simulink model "abs_CS9_LDM_w_EBRDBR"  (Simulink 9.2)
settings: Solver=FixedStepAuto  StartTime=0  StopTime=20  FixedStep=0.0005  RelTol=1e-3  AbsTol=1e-6
values from neighbouring files (symbols this model uses):
  K_Cntr_HiSpd_u8 = 10.0    [DBR_V002.sldd]
  K_Cntr_LowSpd_u8 = 10.0    [DBR_V002.sldd]
  K_Cntr_NrmlSpd_u8 = 10.0    [DBR_V002.sldd]
  K_Cntr_Sdstl_u8 = 10.0    [DBR_V002.sldd]
  K_CSTCtol_ramp_lower = -800.0    [DBR_V002.sldd]
  K_CSTCtol_ramp_upper = 800.0    [DBR_V002.sldd]
  K_DBR_aDBRCSTminDecel = 100.0    [DBR_V002.sldd]
  K_DBR_aDBRDecelEmgHigh_CST_u16 = 500.0    [DBR_V002.sldd]
  K_DBR_aDBRDecelSftLow_CST_u16 = 200.0    [DBR_V002.sldd]
  K_DBR_aDBRDecelStdlstlDegdlvl1_u16 = 600.0    [DBR_V002.sldd]
  K_DBR_aDBRDecelStdlstlDegdlvl2_u16 = 1200.0    [DBR_V002.sldd]
  K_DBR_blCSTSwch_bl = 0.0    [DBR_V002.sldd]
  K_DBR_coDBRDecelFactor1 = 5.0    [DBR_V002.sldd]
  K_DBR_coDBRDecelFactor2 = 3.0    [DBR_V002.sldd]
  K_DBR_lenDBRStdlstlDegdlvl_u16 = 1800.0    [DBR_V002.sldd]
  K_DBR_velCSTPdlDistSpdLmt_s16 = 100.0    [DBR_V002.sldd]
  K_DBR_velDBRCSTlowVehSpd_u16 = 8.0    [DBR_V002.sldd]
  K_DBR_velVehSpdLow_CST_s16 = 14.0    [DBR_V002.sldd]
  K_EBR_aACCHold_flat_u16 = 200.0    [DBR_V002.sldd]
  K_EBR_ACC_ramp_lower = -800.0    [DBR_V002.sldd]
  K_EBR_ACC_ramp_upper = 800.0    [DBR_V002.sldd]
  K_EBR_ACCSBDeclEterDecl_u16 = 200.0    [DBR_V002.sldd]
  K_EBR_ACCSBDeclSlope = 1.0    [DBR_V002.sldd]
  K_EBR_ACCSBminDecl = 100.0    [DBR_V002.sldd]
  K_EBR_velACCVehSpdHiLim_u16 = 431.0    [DBR_V002.sldd]
  K_EBR_velACCVehSpdLim_buffer = 1.0    [DBR_V002.sldd]
  K_EBR_velACCVehSpdLoLim_u16 = 14.0    [DBR_V002.sldd]
  W_EBR_velACCSBEntrVehSpd_u16 = 0.0    [DBR_V002.sldd]
undefined symbols (not defined in the file or in its folder): sigbuilder_block
libraries: simulink x8, LDM_Controller x2, Solver_SF x1
(part 1 of 2)
settings Model: DataDictionary=totalDataDict.sldd  Creator=ywata  LastModifiedBy=wxmjy  PauseTimes=12.5  NumberOfSteps=10  ExtModeTrigMode=oneshot  ExtModeArmWhenConnect=off
settings SolverCC: AutoScaleAbsTol=off
settings DataIOCC: LimitDataPoints=off  SaveFormat=Dataset  SignalLoggingSaveFormat=Dataset  SignalLoggingName=sigsOut
settings OptimizationCC: BlockReduction=off  BooleanDataType=off  ExpressionDepthLimit=2147483647
settings DebuggingCC: SaveWithParameterizedLinksMsg=none  SignalResolutionControl=TryResolveAllWithWarning  MultiTaskDSMMsg=warning  MultiTaskCondExecSysMsg=none
settings HardwareCC: TargetUnknown=on
settings RTWCC: TemplateMakefile=grt_vc.tmf
settings GRTTargetCC: TargetFcnLib=ansi_tfl_tmw.mat  GeneratePreprocessorConditionals=Use local settings
settings ConfigComp: CovHtmlReporting=off

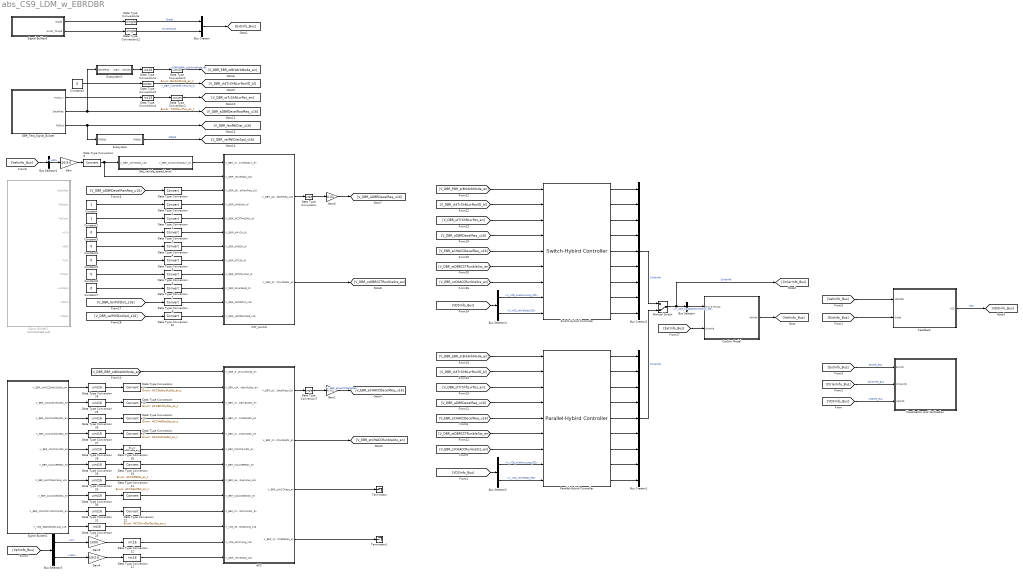
== system abs_CS9_LDM_w_EBRDBR ==
  ACC : Subsystem
  Bus Creator : BusCreator  Inputs=2
  Bus Creator1 : BusCreator  Inputs=9
  Bus Creator2 : BusCreator  Inputs=9
  Bus Selector : BusSelector  OutputSignals=V_LDM_torqDecelCtrlerOut_f32
  Bus Selector1 : BusSelector  OutputSignals=xdot
  Bus Selector2 : BusSelector  OutputSignals=V_VDS_aVehAccLong_f32,V_VDS_velVehSpd_f32
  Bus Selector3 : BusSelector  OutputSignals=ax,xdot
  Bus Selector4 : BusSelector  OutputSignals=V_VDS_aVehAccLong_f32,V_VDS_velVehSpd_f32
  CST_control : Subsystem
  CarSim Model : Subsystem
  Constant : Constant
  Constant1 : Constant
  Constant{2..7} (6 alike) : Constant  Value=0
  DBR_Test_Signal_Builder : Subsystem  Tag=STV Subsys  LoadFcn=sigbuilder_block('load',[245.25 59.25 620.25 643.5 ]);  StartFcn=sigbuilder_block('start');  StopFcn=sigbuilder_block('stop');  ClipboardFcn=sigbuilder_block('clipboard');  mask(Sigbuilder block){tuvar=[0:10]}
      mask help: Simulink:masks:SigbuilderBlock_MD
      mask init:
      | if ~strcmp(get_param(bdroot(gcbh),'SimulationStatus'),'stopped') tuvar = sigbuilder_block('maskInit'); end
      settings: CopyFcn=sigbuilder_block('copy');  DeleteFcn=sigbuilder_block('delete');  ModelCloseFcn=sigbuilder_block('modelClose');  PreSaveFcn=sigbuilder_block('preSave');  PauseFcn=sigbuilder_block('pause');  ContinueFcn=sigbuilder_block('continue');  NameChangeFcn=sigbuilder_block('namechange');  OpenFcn=sigbuilder_block('open',[782.25 67.5 620.25 643.5 ]);  CloseFcn=sigbuilder_block('close');
      mask Display: plot(0, 0, 100, 100,[2, 2, 32, 32, 2], [68, 8, 8, 68, 68],[32, 2], [38, 38], [32, 19, 2],[53, 60, 44], [32, 17, 17, 2],[16, 16, 31, 31]);txt = getActiveGroup(gcbh);text(2, 100, txt,'verticalAlignment', 'top');
  Data Type  Conversion{,6..7,12} (4 alike) : DataTypeConversion  OutDataTypeStr=single
  Data Type  Conversion1 : DataTypeConversion  OutDataTypeStr=Enum: BrkArbMode_en_t
  Data Type  Conversion2 : DataTypeConversion  OutDataTypeStr=Enum: TrShftLvrPos_en_t
  Data Type  Conversion3 : DataTypeConversion  OutDataTypeStr=int16
  Data Type  Conversion4 : DataTypeConversion  OutDataTypeStr=int16
  Data Type  Conversion5 : DataTypeConversion  OutDataTypeStr=boolean  RndMeth=Nearest
  Data Type Conversion{,1..8,32} (10 alike) : DataTypeConversion
  Data Type Conversion11 : DataTypeConversion  OutDataTypeStr=int16  RndMeth=Ceiling
  Data Type Conversion12 : DataTypeConversion  OutDataTypeStr=int16  RndMeth=Ceiling
  Data Type Conversion14 : DataTypeConversion  OutDataTypeStr=Enum: ACCStdbySkpSts_en_t
  Data Type Conversion15 : DataTypeConversion  OutDataTypeStr=Enum: ACCBrkSkpSts_en_t
  Data Type Conversion16 : DataTypeConversion  OutDataTypeStr=Enum: ACCHldSkpSts_en_t
  Data Type Conversion17 : DataTypeConversion  OutDataTypeStr=Enum: ACCFalCseSts_en_t
  Data Type Conversion18 : DataTypeConversion  OutDataTypeStr=Enum: ACCSysSts_en_t
  Data Type Conversion19 : DataTypeConversion  OutDataTypeStr=Enum: ACCEPBSts_en_t
  Data Type Conversion{20,24..31} (9 alike) : DataTypeConversion  OutDataTypeStr=uint16
  Data Type Conversion21 : DataTypeConversion  OutDataTypeStr=Enum: ACCSebltSts_en_t
  Data Type Conversion22 : DataTypeConversion  OutDataTypeStr=Enum: ACCDrvrDorOpnSts_en_t
  Data Type Conversion23 : DataTypeConversion  OutDataTypeStr=int16
  Data Type Conversion9 : DataTypeConversion  RndMeth=Ceiling
  Feedback : Subsystem
  Gain : Gain  Gain=10/3.6
  Gain1 : Gain  Gain=0.01  OutDataTypeStr=Inherit: Inherit via back propagation
  Gain4 : Gain  Gain=10/3.6
  Gain5 : Gain  Gain=1000
  Gain6 : Gain  Gain=0.01  OutDataTypeStr=Inherit: Inherit via back propagation
  Get_vehicle_speed_level : Subsystem
  Manual Switch : ManualSwitch  CurrentSetting=0
  Parallel-Hybird Controller : LDM_Controller/Parallel-Hybird Controller  SystemSampleTime=-1
  Signal Builder1 : Subsystem  Tag=STV Subsys  Commented=on  LoadFcn=sigbuilder_block('load');  StartFcn=sigbuilder_block('start');  StopFcn=sigbuilder_block('stop');  ClipboardFcn=sigbuilder_block('clipboard');  mask(Sigbuilder block){tuvar=[0:10]}
      mask help: Simulink:masks:SigbuilderBlock_MD
      mask init:
      | if ~strcmp(get_param(bdroot(gcbh),'SimulationStatus'),'stopped') tuvar = sigbuilder_block('maskInit'); end
      settings: CopyFcn=sigbuilder_block('copy');  DeleteFcn=sigbuilder_block('delete');  ModelCloseFcn=sigbuilder_block('modelClose');  PreSaveFcn=sigbuilder_block('preSave');  PauseFcn=sigbuilder_block('pause');  ContinueFcn=sigbuilder_block('continue');  NameChangeFcn=sigbuilder_block('namechange');  OpenFcn=sigbuilder_block('open',[0.75 30.75 718.5 714.75 ]);  CloseFcn=sigbuilder_block('close');
      mask Display: plot(0, 0, 100, 100,[2, 2, 32, 32, 2], [68, 8, 8, 68, 68],[32, 2], [38, 38], [32, 19, 2],[53, 60, 44], [32, 17, 17, 2],[16, 16, 31, 31]);txt = getActiveGroup(gcbh);text(2, 100, txt,'verticalAlignment', 'top');
  Signal Builder2 : Subsystem  Tag=STV Subsys  LoadFcn=sigbuilder_block('load');  StartFcn=sigbuilder_block('start');  StopFcn=sigbuilder_block('stop');  ClipboardFcn=sigbuilder_block('clipboard');  mask(Sigbuilder block){tuvar=[0:10]}
      mask help: Simulink:masks:SigbuilderBlock_MD
      mask init:
      | if ~strcmp(get_param(bdroot(gcbh),'SimulationStatus'),'stopped') tuvar = sigbuilder_block('maskInit'); end
      settings: CopyFcn=sigbuilder_block('copy');  DeleteFcn=sigbuilder_block('delete');  ModelCloseFcn=sigbuilder_block('modelClose');  PreSaveFcn=sigbuilder_block('preSave');  PauseFcn=sigbuilder_block('pause');  ContinueFcn=sigbuilder_block('continue');  NameChangeFcn=sigbuilder_block('namechange');  OpenFcn=sigbuilder_block('open',[0.75 30.75 718.5 714.75 ]);  CloseFcn=sigbuilder_block('close');
      mask Display: plot(0, 0, 100, 100,[2, 2, 32, 32, 2], [68, 8, 8, 68, 68],[32, 2], [38, 38], [32, 19, 2],[53, 60, 44], [32, 17, 17, 2],[16, 16, 31, 31]);txt = getActiveGroup(gcbh);text(2, 100, txt,'verticalAlignment', 'top');
  Signal Builder3 : Subsystem  Tag=STV Subsys  LoadFcn=sigbuilder_block('load');  StartFcn=sigbuilder_block('start');  StopFcn=sigbuilder_block('stop');  ClipboardFcn=sigbuilder_block('clipboard');  mask(Sigbuilder block){tuvar=[0:10]}
      mask help: Simulink:masks:SigbuilderBlock_MD
      mask init:
      | if ~strcmp(get_param(bdroot(gcbh),'SimulationStatus'),'stopped') tuvar = sigbuilder_block('maskInit'); end
      settings: CopyFcn=sigbuilder_block('copy');  DeleteFcn=sigbuilder_block('delete');  ModelCloseFcn=sigbuilder_block('modelClose');  PreSaveFcn=sigbuilder_block('preSave');  PauseFcn=sigbuilder_block('pause');  ContinueFcn=sigbuilder_block('continue');  NameChangeFcn=sigbuilder_block('namechange');  OpenFcn=sigbuilder_block('open',[782.25 67.5 620.25 643.5 ]);  CloseFcn=sigbuilder_block('close');
      mask Display: plot(0, 0, 100, 100,[2, 2, 32, 32, 2], [68, 8, 8, 68, 68],[32, 2], [38, 38], [32, 19, 2],[53, 60, 44], [32, 17, 17, 2],[16, 16, 31, 31]);txt = getActiveGroup(gcbh);text(2, 100, txt,'verticalAlignment', 'top');
  Subsystem : Subsystem
  Subsystem1 : Subsystem
  Switch-Hybird Controller : LDM_Controller/Switch-Hybird Controller  SystemSampleTime=-1
  Terminator : Terminator
  Terminator1 : Terminator
  Visualization and Verification : Subsystem
  wires:
  [ExtInfo_Bus] -> Visualization and Verification/1(ExtInfo)  "ExtInfo_Bus"
  [V_EBR_aCHACCDecelReq_u16] -> Parallel-Hybird Controller/5
  Data Type  Conversion12/1 -> Bus Creator/2  "DriveTorque"
  Data Type  Conversion3/1 -> Data Type  Conversion1/1
  Data Type  Conversion4/1 -> Data Type  Conversion2/1
  [V_EBR_stCHACCRunbleSts_en] -> Parallel-Hybird Controller/7
  Constant2/1 -> Data Type  Conversion5/1
  Data Type  Conversion6/1 -> Bus Creator/1  "Grade"
  Subsystem1/1(stBrkArbMode) -> Data Type  Conversion3/1
  Data Type  Conversion1/1 -> [V_DBR_EBR_stBrkArbMode_en]  "V_DBR_EBR_stBrkArbMode_en"
  DBR_Test_Signal_Builder/1(TrShtLvr) -> Data Type  Conversion4/1
  Data Type  Conversion2/1 -> [V_DBR_stTrShftLvrPos_en]
  Feedback/1(VDS) -> [VDSInfo_Bus]  "VDS"
  Signal Builder3/2(Accel_Torque) -> Data Type  Conversion12/1
  [CtrlerInfo_Bus] -> Visualization and Verification/2(CtrlerInfo)  "CtrlerInfo_Bus"
  Data Type  Conversion5/1 -> [V_DBR_vldTrShftLvrPosVD_bl]  "V_DBR_vldTrShftLvrPosVD_bl"
  [VehInfo_Bus] -> Feedback/1(VehFdbk)
  CarSim Model/1(VehInfo) -> [VehInfo_Bus]
  Bus Creator/1 -> [ExtInfo_Bus]
  Manual Switch/1 -> [CtrlerInfo_Bus], Bus Selector/1  "CtrlerInfo"
  [VDSInfo_Bus] -> Visualization and Verification/3(VehInfo)  "VDSInfo_Bus"
  [ExtInfo_Bus] -> Feedback/2(Grade)
  Bus Selector1/1 -> Gain/1  "<xdot>"
  Get_vehicle_speed_level/1(V_EBR_stACCVehSpdLvl_en) -> CST_control/1(V_EBR_stACCVehSpdLvl_en)
  [V_DBR_aDBRDecelRawReq_u16] -> Data Type Conversion/1
  Constant/1 -> Data Type Conversion1/1
  Constant1/1 -> Data Type Conversion2/1
  Constant3/1 -> Data Type Conversion3/1
  Constant4/1 -> Data Type Conversion4/1
  Constant5/1 -> Data Type Conversion5/1
  Constant6/1 -> Data Type Conversion6/1
  Constant7/1 -> Data Type Conversion7/1
  [VehInfo_Bus] -> Bus Selector1/1
  Data Type Conversion/1 -> CST_control/3(V_DBR_aDBRDecelRawReq_u16)
  Data Type Conversion1/1 -> CST_control/4(V_DBR_stPdlAply_bl)
  Data Type Conversion2/1 -> CST_control/5(V_DBR_blCSTPreCdtin_bl)
  Data Type Conversion3/1 -> CST_control/6(V_DBR_blAYCA_bl)
  Data Type Conversion4/1 -> CST_control/7(V_DBR_blABSA_bl)
  Data Type Conversion5/1 -> CST_control/8(V_DBR_blTCSA_bl)
  Data Type Conversion6/1 -> CST_control/9(V_DBR_blCSTSysFail_bl)
  Data Type Conversion7/1 -> CST_control/10(V_DBR_blLosDecel_bl)
  Data Type Conversion8/1 -> CST_control/11(V_DBR_lenPdlDist_s16)
  Data Type Conversion9/1 -> CST_control/2(V_DBR_velVehSpd_s16), Get_vehicle_speed_level/1(V_DBR_velVehSpd_s16)
  Gain/1 -> Data Type Conversion9/1
  Gain6/1 -> [V_DBR_aDBRDecelReq_u16]
  CST_control/2(V_DBR_stDBRCSTRunbleSts_en) -> [V_DBR_stDBRCSTRunbleSts_en]
  ACC/3(V_EBR_stACCResp_en) -> Terminator/1
  Data Type Conversion11/1 -> ACC/13(V_DBR_velVehSpd_s16)
  ACC/4(V_EBR_stCHACCEPBReq_en) -> Terminator1/1
  [V_DBR_EBR_stBrkArbMode_en] -> ACC/1(V_DBR_EBR_stBrkArbMode_en)
  Gain4/1 -> Data Type Conversion11/1
  [VehInfo_Bus] -> Bus Selector3/1
  Bus Selector3/2 -> Gain4/1  "<xdot>"
  Bus Selector3/1 -> Gain5/1  "<ax>"
  Gain5/1 -> Data Type Conversion12/1
  Data Type Conversion12/1 -> ACC/12(V_VDS_aACCLong_s16)
  ACC/2(V_EBR_stCHACCRunbleSts_en) -> [V_EBR_stCHACCRunbleSts_en]
  Signal Builder2/1(V_EBR_stACCStdbySkpSts_en) -> Data Type Conversion24/1
  Signal Builder2/2(V_EBR_stACCBrkSkpSts_en) -> Data Type Conversion25/1
  Signal Builder2/3(V_EBR_stACCHldSkpSts_en) -> Data Type Conversion26/1
  Signal Builder2/4(V_EBR_stACCFalCseSts_en) -> Data Type Conversion27/1
  Signal Builder2/5(V_EBR_stACCSysSts_en) -> Data Type Conversion28/1
  Signal Builder2/6(V_EBR_stACCEPBSts_en) -> Data Type Conversion29/1
  Signal Builder2/7(V_EBR_aACCReqValue_u16) -> Data Type Conversion20/1
  Signal Builder2/8(V_EBR_stACCSebltSts_en) -> Data Type Conversion30/1
  Signal Builder2/9(V_EBR_stACCDrvrDorOpnSts_en) -> Data Type Conversion31/1
  Signal Builder2/10(V_VDS_degRdSlopeLong_s16) -> Data Type Conversion23/1
  Data Type Conversion14/1 -> ACC/2(V_EBR_stACCStdbySkpSts_en)
  Data Type Conversion15/1 -> ACC/3(V_EBR_stACCBrkSkpSts_en)
  Data Type Conversion16/1 -> ACC/4(V_EBR_stACCHldSkpSts_en)
  Data Type Conversion17/1 -> ACC/5(V_EBR_stACCFalCseSts_en)
  Data Type Conversion18/1 -> ACC/6(V_EBR_stACCSysSts_en)
  Data Type Conversion19/1 -> ACC/7(V_EBR_stACCEPBSts_en)
  Data Type Conversion20/1 -> ACC/8(V_EBR_aACCReqValue_u16)
  Data Type Conversion21/1 -> ACC/9(V_EBR_stACCSebltSts_en)
  Data Type Conversion22/1 -> ACC/10(V_EBR_stACCDrvrDorOpnSts_en)
  Data Type Conversion23/1 -> ACC/11(V_VDS_degRdSlopeLong_s16)
  Data Type Conversion24/1 -> Data Type Conversion14/1
  Data Type Conversion25/1 -> Data Type Conversion15/1
  Data Type Conversion26/1 -> Data Type Conversion16/1
  Data Type Conversion27/1 -> Data Type Conversion17/1
  Data Type Conversion28/1 -> Data Type Conversion18/1
  Data Type Conversion29/1 -> Data Type Conversion19/1
  Data Type Conversion30/1 -> Data Type Conversion21/1
  Data Type Conversion31/1 -> Data Type Conversion22/1
  Data Type Conversion32/1 -> CST_control/12(V_DBR_velPdlDistSpd_s16)
  [V_DBR_aDBRDecelReq_u16] -> Parallel-Hybird Controller/4
  [V_DBR_stDBRCSTRunbleSts_en] -> Parallel-Hybird Controller/6
  [V_DBR_EBR_stBrkArbMode_en] -> Parallel-Hybird Controller/1
  [V_DBR_vldTrShftLvrPosVD_bl] -> Parallel-Hybird Controller/2
  [V_DBR_stTrShftLvrPos_en] -> Parallel-Hybird Controller/3
  Bus Selector/1 -> CarSim Model/1(Brake Torque)  "<V_LDM_torqDecelCtrlerOut_f32>"
  DBR_Test_Signal_Builder/2(DecelReq) -> Subsystem1/1(DecelReq), [V_DBR_aDBRDecelRawReq_u16]
  DBR_Test_Signal_Builder/3(PldDist) -> Subsystem/1(PldDist), [V_DBR_lenPdlDist_s16]
  Subsystem/1(PldSpd) -> [V_DBR_velPdlDistSpd_s16]  "PldSpd"
  [V_DBR_velPdlDistSpd_s16] -> Data Type Conversion32/1
  [V_DBR_lenPdlDist_s16] -> Data Type Conversion8/1
  Signal Builder3/1(Grade) -> Data Type  Conversion6/1
  [VDSInfo_Bus] -> Bus Selector2/1
  Bus Selector2/1 -> Parallel-Hybird Controller/8  "<V_VDS_aVehAccLong_f32>"
  Bus Selector2/2 -> Parallel-Hybird Controller/9  "<V_VDS_velVehSpd_f32>"
  Parallel-Hybird Controller/1 -> Bus Creator1/1
  Parallel-Hybird Controller/2 -> Bus Creator1/2
  Parallel-Hybird Controller/4 -> Bus Creator1/4
  Parallel-Hybird Controller/5 -> Bus Creator1/5
  Parallel-Hybird Controller/6 -> Bus Creator1/6
  Parallel-Hybird Controller/7 -> Bus Creator1/7
  Parallel-Hybird Controller/8 -> Bus Creator1/8
  Bus Selector4/2 -> Switch-Hybird Controller/9  "<V_VDS_velVehSpd_f32>"
  Bus Selector4/1 -> Switch-Hybird Controller/8  "<V_VDS_aVehAccLong_f32>"
  [VDSInfo_Bus] -> Bus Selector4/1
  [V_DBR_stTrShftLvrPos_en] -> Switch-Hybird Controller/3
  [V_DBR_vldTrShftLvrPosVD_bl] -> Switch-Hybird Controller/2
  [V_DBR_EBR_stBrkArbMode_en] -> Switch-Hybird Controller/1
  [V_DBR_stDBRCSTRunbleSts_en] -> Switch-Hybird Controller/6
  [V_DBR_aDBRDecelReq_u16] -> Switch-Hybird Controller/4
  [V_EBR_stCHACCRunbleSts_en] -> Switch-Hybird Controller/7
  [V_EBR_aCHACCDecelReq_u16] -> Switch-Hybird Controller/5
  Switch-Hybird Controller/8 -> Bus Creator2/8
  Switch-Hybird Controller/7 -> Bus Creator2/7
  Switch-Hybird Controller/6 -> Bus Creator2/6
  Switch-Hybird Controller/5 -> Bus Creator2/5
  Switch-Hybird Controller/4 -> Bus Creator2/4
  Switch-Hybird Controller/2 -> Bus Creator2/2
  Switch-Hybird Controller/1 -> Bus Creator2/1
  Bus Creator2/1 -> Manual Switch/1  "CtrlerInfo"
  Bus Creator1/1 -> Manual Switch/2  "CtrlerInfo"
  Switch-Hybird Controller/9 -> Bus Creator2/9
  Parallel-Hybird Controller/9 -> Bus Creator1/9
  [ExtInfo_Bus] -> CarSim Model/2(throttle)
  Parallel-Hybird Controller/3 -> Bus Creator1/3
  Switch-Hybird Controller/3 -> Bus Creator2/3
  Data Type  Conversion7/1 -> Gain1/1
  Data Type  Conversion/1 -> Gain6/1
  CST_control/1(V_DBR_aDBRDecelReq_u16) -> Data Type  Conversion/1
  Gain1/1 -> [V_EBR_aCHACCDecelReq_u16]  "V_EBR_aCHACCDecelReq"
  ACC/1(V_EBR_aCHACCDecelReq_u16) -> Data Type  Conversion7/1

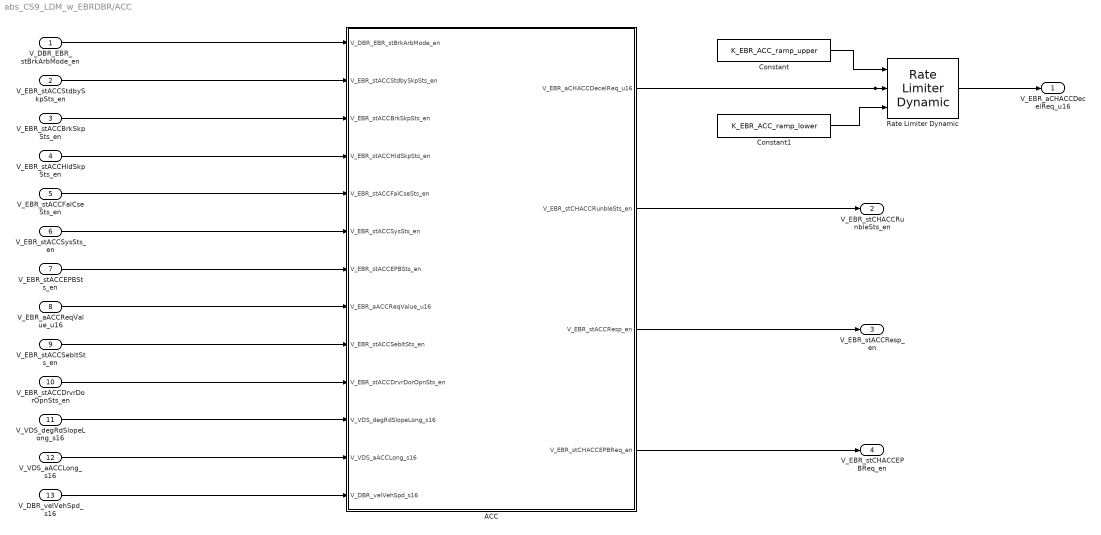
== system abs_CS9_LDM_w_EBRDBR/ACC ==
  V_DBR_EBR_stBrkArbMode_en : Inport
  V_EBR_stACCStdbySkpSts_en : Inport  Port=2
  V_EBR_stACCBrkSkpSts_en : Inport  Port=3
  V_EBR_stACCHldSkpSts_en : Inport  Port=4
  V_EBR_stACCFalCseSts_en : Inport  Port=5
  V_EBR_stACCSysSts_en : Inport  Port=6
  V_EBR_stACCEPBSts_en : Inport  Port=7
  V_EBR_aACCReqValue_u16 : Inport  Port=8
  V_EBR_stACCSebltSts_en : Inport  Port=9
  V_EBR_stACCDrvrDorOpnSts_en : Inport  Port=10
  V_VDS_degRdSlopeLong_s16 : Inport  Port=11
  V_VDS_aACCLong_s16 : Inport  Port=12
  V_DBR_velVehSpd_s16 : Inport  Port=13
  ACC : Stateflow chart  TreatAsAtomicUnit=on
  Constant : Constant  Value=K_EBR_ACC_ramp_upper
  Constant1 : Constant  Value=K_EBR_ACC_ramp_lower
  Rate Limiter Dynamic : simulink/Discontinuities/Rate Limiter Dynamic
      settings: SourceProductName=Simulink
  V_EBR_aCHACCDecelReq_u16 : Outport
  V_EBR_stCHACCRunbleSts_en : Outport  Port=2  OutDataTypeStr=Enum: CHACCRunbleSts_en_t
  V_EBR_stACCResp_en : Outport  Port=3  OutDataTypeStr=Enum: ACCResp_en_t
  V_EBR_stCHACCEPBReq_en : Outport  Port=4  OutDataTypeStr=Enum: CHACCEPBReq_en_t
  wires:
  V_EBR_stACCStdbySkpSts_en/1 -> ACC/2(V_EBR_stACCStdbySkpSts_en)
  V_EBR_stACCBrkSkpSts_en/1 -> ACC/3(V_EBR_stACCBrkSkpSts_en)
  V_EBR_stACCHldSkpSts_en/1 -> ACC/4(V_EBR_stACCHldSkpSts_en)
  V_EBR_stACCFalCseSts_en/1 -> ACC/5(V_EBR_stACCFalCseSts_en)
  V_EBR_stACCSysSts_en/1 -> ACC/6(V_EBR_stACCSysSts_en)
  V_EBR_stACCEPBSts_en/1 -> ACC/7(V_EBR_stACCEPBSts_en)
  V_EBR_aACCReqValue_u16/1 -> ACC/8(V_EBR_aACCReqValue_u16)
  V_DBR_EBR_stBrkArbMode_en/1 -> ACC/1(V_DBR_EBR_stBrkArbMode_en)
  V_EBR_stACCSebltSts_en/1 -> ACC/9(V_EBR_stACCSebltSts_en)
  V_EBR_stACCDrvrDorOpnSts_en/1 -> ACC/10(V_EBR_stACCDrvrDorOpnSts_en)
  V_VDS_degRdSlopeLong_s16/1 -> ACC/11(V_VDS_degRdSlopeLong_s16)
  V_VDS_aACCLong_s16/1 -> ACC/12(V_VDS_aACCLong_s16)
  V_DBR_velVehSpd_s16/1 -> ACC/13(V_DBR_velVehSpd_s16)
  ACC/2(V_EBR_stCHACCRunbleSts_en) -> V_EBR_stCHACCRunbleSts_en/1
  ACC/3(V_EBR_stACCResp_en) -> V_EBR_stACCResp_en/1
  ACC/4(V_EBR_stCHACCEPBReq_en) -> V_EBR_stCHACCEPBReq_en/1
  Constant1/1 -> Rate Limiter Dynamic/3
  Constant/1 -> Rate Limiter Dynamic/1
  ACC/1(V_EBR_aCHACCDecelReq_u16) -> Rate Limiter Dynamic/2, V_EBR_aCHACCDecelReq_u16/1

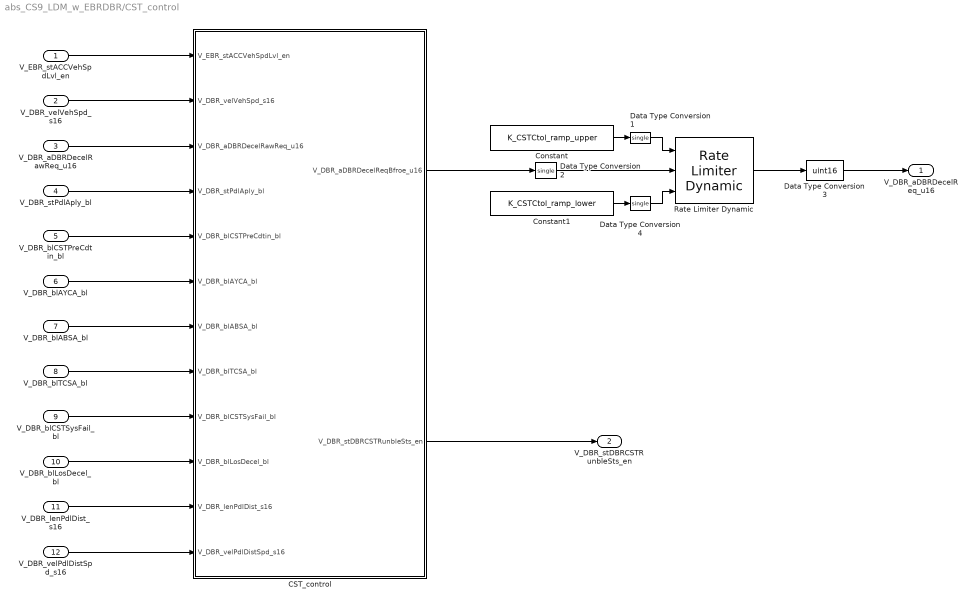
== system abs_CS9_LDM_w_EBRDBR/CST_control ==
  V_EBR_stACCVehSpdLvl_en : Inport
  V_DBR_velVehSpd_s16 : Inport  Port=2
  V_DBR_aDBRDecelRawReq_u16 : Inport  Port=3
  V_DBR_stPdlAply_bl : Inport  Port=4
  V_DBR_blCSTPreCdtin_bl : Inport  Port=5
  V_DBR_blAYCA_bl : Inport  Port=6
  V_DBR_blABSA_bl : Inport  Port=7
  V_DBR_blTCSA_bl : Inport  Port=8
  V_DBR_blCSTSysFail_bl : Inport  Port=9
  V_DBR_blLosDecel_bl : Inport  Port=10
  V_DBR_lenPdlDist_s16 : Inport  Port=11
  V_DBR_velPdlDistSpd_s16 : Inport  Port=12
  CST_control : Stateflow chart  TreatAsAtomicUnit=on
  Constant : Constant  Value=K_CSTCtol_ramp_upper
  Constant1 : Constant  Value=K_CSTCtol_ramp_lower
  Data Type Conversion1 : DataTypeConversion  OutDataTypeStr=single
  Data Type Conversion2 : DataTypeConversion  OutDataTypeStr=single
  Data Type Conversion3 : DataTypeConversion  OutDataTypeStr=uint16
  Data Type Conversion4 : DataTypeConversion  OutDataTypeStr=single
  Rate Limiter Dynamic : simulink/Discontinuities/Rate Limiter Dynamic
  V_DBR_aDBRDecelReq_u16 : Outport
  V_DBR_stDBRCSTRunbleSts_en : Outport  Port=2
  wires:
  V_EBR_stACCVehSpdLvl_en/1 -> CST_control/1(V_EBR_stACCVehSpdLvl_en)
  V_DBR_velVehSpd_s16/1 -> CST_control/2(V_DBR_velVehSpd_s16)
  V_DBR_aDBRDecelRawReq_u16/1 -> CST_control/3(V_DBR_aDBRDecelRawReq_u16)
  V_DBR_stPdlAply_bl/1 -> CST_control/4(V_DBR_stPdlAply_bl)
  V_DBR_blCSTPreCdtin_bl/1 -> CST_control/5(V_DBR_blCSTPreCdtin_bl)
  V_DBR_blAYCA_bl/1 -> CST_control/6(V_DBR_blAYCA_bl)
  V_DBR_blABSA_bl/1 -> CST_control/7(V_DBR_blABSA_bl)
  V_DBR_blTCSA_bl/1 -> CST_control/8(V_DBR_blTCSA_bl)
  V_DBR_blCSTSysFail_bl/1 -> CST_control/9(V_DBR_blCSTSysFail_bl)
  V_DBR_blLosDecel_bl/1 -> CST_control/10(V_DBR_blLosDecel_bl)
  V_DBR_lenPdlDist_s16/1 -> CST_control/11(V_DBR_lenPdlDist_s16)
  CST_control/2(V_DBR_stDBRCSTRunbleSts_en) -> V_DBR_stDBRCSTRunbleSts_en/1
  Rate Limiter Dynamic/1 -> Data Type Conversion3/1
  CST_control/1(V_DBR_aDBRDecelReqBfroe_u16) -> Data Type Conversion2/1
  Data Type Conversion1/1 -> Rate Limiter Dynamic/1
  Data Type Conversion4/1 -> Rate Limiter Dynamic/3
  Data Type Conversion2/1 -> Rate Limiter Dynamic/2
  Constant/1 -> Data Type Conversion1/1
  Constant1/1 -> Data Type Conversion4/1
  Data Type Conversion3/1 -> V_DBR_aDBRDecelReq_u16/1
  V_DBR_velPdlDistSpd_s16/1 -> CST_control/12(V_DBR_velPdlDistSpd_s16)

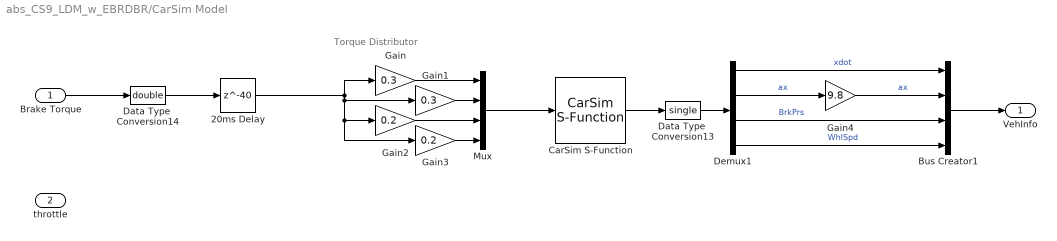
== system abs_CS9_LDM_w_EBRDBR/CarSim Model ==
  note: Torque Distributor
  Brake Torque : Inport
  throttle : Inport  Port=2
  20ms Delay : Delay  DelayLength=40
  Bus Creator1 : BusCreator  Inputs=4
  CarSim S-Function : Solver_SF/CarSim S-Function  Priority=1  SIMFILE=simfile.sim  Run_RTs=off  vs_state_ind=Run  StopMode_ind=Vehicle Model
  Data Type  Conversion13 : DataTypeConversion  OutDataTypeStr=single
  Data Type  Conversion14 : DataTypeConversion  OutDataTypeStr=double
  Demux1 : Demux  Outputs=[1 1 4 4]
  Gain : Gain  Gain=0.3
  Gain1 : Gain  Gain=0.3
  Gain2 : Gain  Gain=0.2
  Gain3 : Gain  Gain=0.2
  Gain4 : Gain  Gain=9.8  OutDataTypeStr=single
  Mux : Mux
  VehInfo : Outport
  wires:
  CarSim S-Function/1 -> Data Type  Conversion13/1
  Bus Creator1/1 -> VehInfo/1
  Demux1/2 -> Gain4/1  "ax"
  Data Type  Conversion13/1 -> Demux1/1
  Demux1/3 -> Bus Creator1/3  "BrkPrs"
  Demux1/4 -> Bus Creator1/4  "WhlSpd"
  Demux1/1 -> Bus Creator1/1  "xdot"
  Brake Torque/1 -> Data Type  Conversion14/1
  Mux/1 -> CarSim S-Function/1
  Gain/1 -> Mux/1
  Gain1/1 -> Mux/2
  Data Type  Conversion14/1 -> 20ms Delay/1
  Gain2/1 -> Mux/3
  Gain3/1 -> Mux/4
  20ms Delay/1 -> Gain3/1, Gain2/1, Gain1/1, Gain/1
  Gain4/1 -> Bus Creator1/2  "ax"

== system abs_CS9_LDM_w_EBRDBR/DBR_Test_Signal_Builder ==
  Demux : Demux  Tag=STV Demux  Outputs=3
  FromWs : FromWorkspace  Tag=STV FromWs  VariableName=tuvar  SampleTime=0  SigBuilderData=DataTag0  VnvData=DataTag1
      SigBuilderData=|
      | common.afterFinalStr = 'Extrapolate'
      | common.sampleTime = 0
      | dataSet(1).timeRange = [0 20]
      | dataSet(1).name = 'DBR_ramp'
      | dataSet(2).timeRange = [0 20]
      | dataSet(2).name = 'DBR_ramp1'
      | dataSet(3).timeRange = [0 20]
      | dataSet(3).name = 'Case1'
      | dataSet(4).timeRange = [0 20]
      | dataSet(4).name = 'Case2'
      | sbobj.Groups(1).Name = 'DBR_ramp'
      | sbobj.Groups(1).Signals(1).Name = 'TrShtLvr'
      | sbobj.Groups(1).Signals(1).XData = [0 20]
      | sbobj.Groups(1).Signals(1).YData = [4 4]
      | sbobj.Groups(1).Signals(2).Name = 'DecelReq'
      | sbobj.Groups(1).Signals(2).XData = [0 4.8 4.8 8.15 8.15 9.85 9.85 14 20]
      | sbobj.Groups(1).Signals(2).YData = [5 5 490 490 180 180 495 0 0]
      | sbobj.Groups(1).Signals(3).Name = 'PldDist'
      | sbobj.Groups(1).Signals(3).XData = [0 2.1 6 10.25 20]
      | sbobj.Groups(1).Signals(3).YData = [0 0 450 0 0]
      | sbobj.Groups(1).TimeRange = [0 20]
      | sbobj.Groups(2).Name = 'DBR_ramp1'
      | sbobj.Groups(2).Signals(1).Name = 'TrShtLvr'
      | sbobj.Groups(2).Signals(1).XData = [0 20]
      | sbobj.Groups(2).Signals(1).YData = [4 4]
      | sbobj.Groups(2).Signals(2).Name = 'DecelReq'
      | sbobj.Groups(2).Signals(2).XData = [0 3.4 3.4 14 14 20]
      | sbobj.Groups(2).Signals(2).YData = [0 0 300 300 20 20]
      | sbobj.Groups(2).Signals(3).Name = 'PldDist'
      | sbobj.Groups(2).Signals(3).XData = [0 20]
      | sbobj.Groups(2).Signals(3).YData = [0 0]
      | sbobj.Groups(2).TimeRange = [0 20]
      | sbobj.Groups(3).Name = 'Case1'
      | sbobj.Groups(3).Signals(1).Name = 'TrShtLvr'
      | sbobj.Groups(3).Signals(1).XData = [0 0.5 3.5 6.5 20]
      | sbobj.Groups(3).Signals(1).YData = [4 4 4 4 4]
      | sbobj.Groups(3).Signals(2).Name = 'DecelReq'
      | sbobj.Groups(3).Signals(2).XData = [0 0.5 3.5 7 12 20]
      | sbobj.Groups(3).Signals(2).YData = [0 0 500 500 0 0]
      | sbobj.Groups(3).Signals(3).Name = 'PldDist'
      | sbobj.Groups(3).Signals(3).XData = [0 0.5 3.5 6.5 20]
      | sbobj.Groups(3).Signals(3).YData = [0 0 50 0 0]
      | sbobj.Groups(3).TimeRange = [0 20]
      | sbobj.Groups(4).Name = 'Case2'
      | sbobj.Groups(4).Signals(1).Name = 'TrShtLvr'
      | sbobj.Groups(4).Signals(1).XData = [0 0.5 1 1.5 20]
      | sbobj.Groups(4).Signals(1).YData = [4 4 4 4 4]
      | sbobj.Groups(4).Signals(2).Name = 'DecelReq'
      | sbobj.Groups(4).Signals(2).XData = [0 0.5 1 1.5 4.9 5.8 7 8.2 9.5 10.35 11.5 12.45 13.7 20]
      | sbobj.Groups(4).Signals(2).YData = [0 0 400 0 0 315 0 0 435 0 0 325 0 0]
      | sbobj.Groups(4).Signals(3).Name = 'PldDist'
      | sbobj.Groups(4).Signals(3).XData = [0 0.5 1 1.5 20]
      | sbobj.Groups(4).Signals(3).YData = [0 0 150 0 0]
      | sbobj.Groups(4).TimeRange = [0 20]
  TrShtLvr : Outport  Tag=STV Outport
  DecelReq : Outport  Tag=STV Outport  Port=2
  PldDist : Outport  Tag=STV Outport  Port=3
  wires:
  FromWs/1 -> Demux/1
  Demux/1 -> TrShtLvr/1
  Demux/2 -> DecelReq/1
  Demux/3 -> PldDist/1

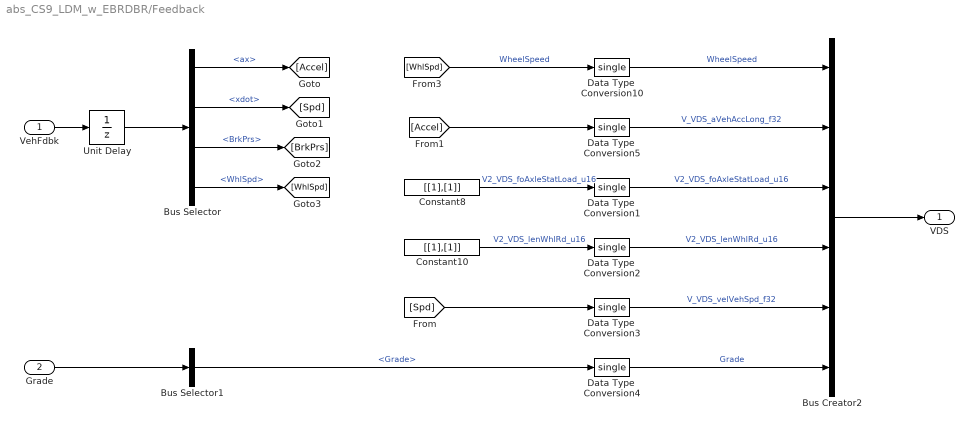
== system abs_CS9_LDM_w_EBRDBR/Feedback ==
  VehFdbk : Inport
  Grade : Inport  Port=2
  Bus Creator2 : BusCreator  Inputs=6
  Bus Selector : BusSelector  OutputSignals=ax,xdot,BrkPrs,WhlSpd
  Bus Selector1 : BusSelector  OutputSignals=Grade
  Constant10 : Constant  Value=[[1],[1]]  OutDataTypeStr=Inherit: Inherit via back propagation
  Constant8 : Constant  Value=[[1],[1]]  OutDataTypeStr=Inherit: Inherit via back propagation
  Data Type  Conversion{1..5,10} (6 alike) : DataTypeConversion  OutDataTypeStr=single
  Unit Delay : UnitDelay  SampleTime=-1
  VDS : Outport
  wires:
  Data Type  Conversion3/1 -> Bus Creator2/5  "V_VDS_velVehSpd_f32"
  Data Type  Conversion10/1 -> Bus Creator2/1  "WheelSpeed"
  Data Type  Conversion2/1 -> Bus Creator2/4  "V2_VDS_lenWhlRd_u16"
  Bus Creator2/1 -> VDS/1
  Data Type  Conversion1/1 -> Bus Creator2/3  "V2_VDS_foAxleStatLoad_u16"
  VehFdbk/1 -> Unit Delay/1
  Bus Selector/1 -> [Accel]  "<ax>"
  Bus Selector/2 -> [Spd]  "<xdot>"
  Bus Selector/3 -> [BrkPrs]  "<BrkPrs>"
  Bus Selector/4 -> [WhlSpd]  "<WhlSpd>"
  Unit Delay/1 -> Bus Selector/1
  Data Type  Conversion4/1 -> Bus Creator2/6  "Grade"
  Constant8/1 -> Data Type  Conversion1/1  "V2_VDS_foAxleStatLoad_u16"
  Constant10/1 -> Data Type  Conversion2/1  "V2_VDS_lenWhlRd_u16"
  Grade/1 -> Bus Selector1/1
  Bus Selector1/1 -> Data Type  Conversion4/1  "<Grade>"
  [WhlSpd] -> Data Type  Conversion10/1  "WheelSpeed"
  [Spd] -> Data Type  Conversion3/1
  [Accel] -> Data Type  Conversion5/1
  Data Type  Conversion5/1 -> Bus Creator2/2  "V_VDS_aVehAccLong_f32"

== system abs_CS9_LDM_w_EBRDBR/Get_vehicle_speed_level ==
  V_DBR_velVehSpd_s16 : Inport  OutDataTypeStr=int16
  Data Type Conversion : DataTypeConversion  OutDataTypeStr=uint16
  Get_vehicle_speed_level : Stateflow chart  TreatAsAtomicUnit=on
  V_EBR_stACCVehSpdLvl_en : Outport
  wires:
  Get_vehicle_speed_level/1(V_EBR_stACCVehSpdLvl_en) -> V_EBR_stACCVehSpdLvl_en/1
  V_DBR_velVehSpd_s16/1 -> Data Type Conversion/1
  Data Type Conversion/1 -> Get_vehicle_speed_level/1(V_DBR_velVehSpd_u16)

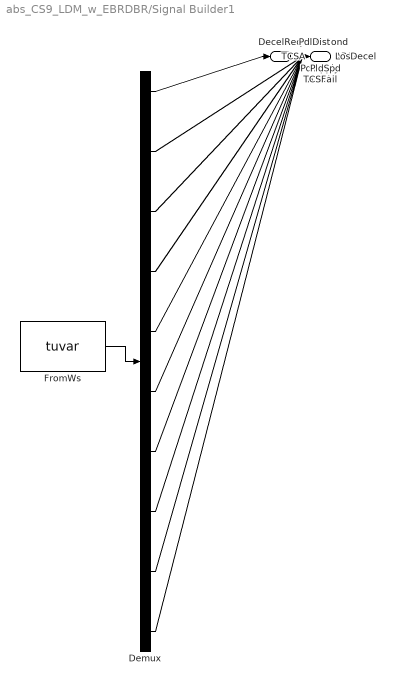
== system abs_CS9_LDM_w_EBRDBR/Signal Builder1 ==
  Demux : Demux  Tag=STV Demux  Outputs=10
  FromWs : FromWorkspace  Tag=STV FromWs  VariableName=tuvar  SampleTime=0  SigBuilderData=DataTag2  VnvData=DataTag3
      SigBuilderData=|
      | common.afterFinalStr = 'Extrapolate'
      | common.sampleTime = 0
      | dataSet.timeRange = [0 20]
      | dataSet.name = 'Group 1'
      | sbobj.Groups.Name = 'Group 1'
      | sbobj.Groups.Signals(1).Name = 'DecelReq'
      | sbobj.Groups.Signals(1).XData = [0 8.1 12 20]
      | sbobj.Groups.Signals(1).YData = [300 370 200 400]
      | sbobj.Groups.Signals(2).Name = 'PdlApply'
      | sbobj.Groups.Signals(2).XData = [0 20]
      | sbobj.Groups.Signals(2).YData = [1 1]
      | sbobj.Groups.Signals(3).Name = 'PreCond'
      | sbobj.Groups.Signals(3).XData = [0 20]
      | sbobj.Groups.Signals(3).YData = [1 1]
      | sbobj.Groups.Signals(4).Name = 'AYCA'
      | sbobj.Groups.Signals(4).XData = [0 20]
      | sbobj.Groups.Signals(4).YData = [0 0]
      | sbobj.Groups.Signals(5).Name = 'ABSA'
      | sbobj.Groups.Signals(5).XData = [0 20]
      | sbobj.Groups.Signals(5).YData = [0 0]
      | sbobj.Groups.Signals(6).Name = 'TCSA'
      | sbobj.Groups.Signals(6).XData = [0 20]
      | sbobj.Groups.Signals(6).YData = [0 0]
      | sbobj.Groups.Signals(7).Name = 'TCSFail'
      | sbobj.Groups.Signals(7).XData = [0 20]
      | sbobj.Groups.Signals(7).YData = [0 0]
      | sbobj.Groups.Signals(8).Name = 'LosDecel'
      | sbobj.Groups.Signals(8).XData = [0 20]
      | sbobj.Groups.Signals(8).YData = [0 0]
      | sbobj.Groups.Signals(9).Name = 'PdlDist'
      | sbobj.Groups.Signals(9).XData = [0 1 5 10 20]
      | sbobj.Groups.Signals(9).YData = [0 0 500 1 1]
      | sbobj.Groups.Signals(10).Name = 'PldSpd'
      | sbobj.Groups.Signals(10).XData = [0 5.4 10 10 20]
      | sbobj.Groups.Signals(10).YData = [0 115 105 1 1]
      | sbobj.Groups.TimeRange = [0 20]
  DecelReq : Outport  Tag=STV Outport
  PdlApply : Outport  Tag=STV Outport  Port=2
  PreCond : Outport  Tag=STV Outport  Port=3
  AYCA : Outport  Tag=STV Outport  Port=4
  ABSA : Outport  Tag=STV Outport  Port=5
  TCSA : Outport  Tag=STV Outport  Port=6
  TCSFail : Outport  Tag=STV Outport  Port=7
  LosDecel : Outport  Tag=STV Outport  Port=8
  PdlDist : Outport  Tag=STV Outport  Port=9
  PldSpd : Outport  Tag=STV Outport  Port=10
  wires:
  FromWs/1 -> Demux/1
  Demux/1 -> DecelReq/1
  Demux/2 -> PdlApply/1
  Demux/3 -> PreCond/1
  Demux/4 -> AYCA/1
  Demux/5 -> ABSA/1
  Demux/6 -> TCSA/1
  Demux/7 -> TCSFail/1
  Demux/8 -> LosDecel/1
  Demux/9 -> PdlDist/1
  Demux/10 -> PldSpd/1

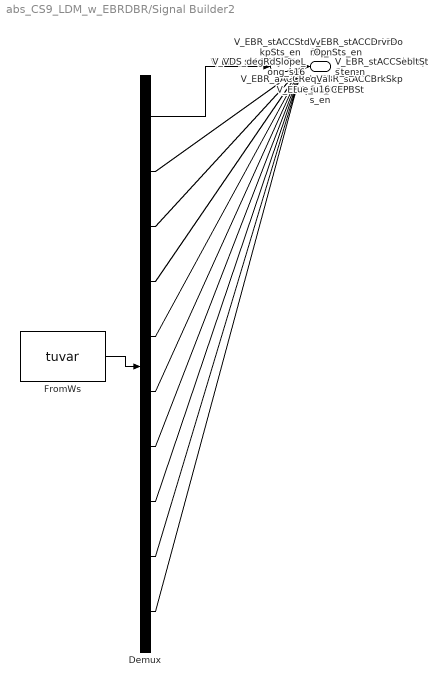
== system abs_CS9_LDM_w_EBRDBR/Signal Builder2 ==
  Demux : Demux  Tag=STV Demux  Outputs=10
  FromWs : FromWorkspace  Tag=STV FromWs  VariableName=tuvar  SampleTime=0  SigBuilderData=DataTag4  VnvData=DataTag5
      SigBuilderData=|
      | common.afterFinalStr = 'Extrapolate'
      | common.sampleTime = 0
      | dataSet.timeRange = [0 36]
      | dataSet.name = 'Sheet1'
      | sbobj.Name = 'Signal Builder'
      | sbobj.Groups.Name = 'Sheet1'
      | sbobj.Groups.Signals(1).Name = 'V_EBR_stACCStdbySkpSts_en'
      | sbobj.Groups.Signals(1).XData = [0 1 1 2 3 10 30 30 31 32 33 35 35 36]
      | sbobj.Groups.Signals(1).YData = [0 0 1 1 1 1 1 2 2 2 2 2 0 0]
      | sbobj.Groups.Signals(2).Name = 'V_EBR_stACCBrkSkpSts_en'
      | sbobj.Groups.Signals(2).XData = [0 1 1 2 3 10 30 30 31 32 33 35 35 36]
      | sbobj.Groups.Signals(2).YData = [0 0 1 1 1 1 1 3 3 3 3 3 0 0]
      | sbobj.Groups.Signals(3).Name = 'V_EBR_stACCHldSkpSts_en'
      | sbobj.Groups.Signals(3).XData = [0 1 1 2 3 10 30 30 31 32 33 35 35 36]
      | sbobj.Groups.Signals(3).YData = [0 0 1 1 1 1 1 3 3 3 3 3 0 0]
      | sbobj.Groups.Signals(4).Name = 'V_EBR_stACCFalCseSts_en'
      | sbobj.Groups.Signals(4).XData = [0 1 2 3 10 30 31 32 33 35 36]
      | sbobj.Groups.Signals(4).YData = [0 0 0 0 0 0 0 0 0 0 0]
      | sbobj.Groups.Signals(5).Name = 'V_EBR_stACCSysSts_en'
      | sbobj.Groups.Signals(5).XData = [0 1 1 2 3 10 30 31 32 33 35 36]
      | sbobj.Groups.Signals(5).YData = [0 0 2 2 2 2 2 2 2 2 2 2]
      | sbobj.Groups.Signals(6).Name = 'V_EBR_stACCEPBSts_en'
      | sbobj.Groups.Signals(6).XData = [0 1 2 3 10 30 31 32 33 35 36]
      | sbobj.Groups.Signals(6).YData = [0 0 0 0 0 0 0 0 0 0 0]
      | sbobj.Groups.Signals(7).Name = 'V_EBR_aACCReqValue_u16'
      | sbobj.Groups.Signals(7).XData = [0 1 1 2 3 10 30 30 31 32 33 35 36]
      | sbobj.Groups.Signals(7).YData = [0 0 300 300 300 300 300 0 0 0 0 0 0]
      | sbobj.Groups.Signals(8).Name = 'V_EBR_stACCSebltSts_en'
      | sbobj.Groups.Signals(8).XData = [0 1 2 3 10 30 31 32 33 35 36]
      | sbobj.Groups.Signals(8).YData = [0 0 0 0 0 0 0 0 0 0 0]
      | sbobj.Groups.Signals(9).Name = 'V_EBR_stACCDrvrDorOpnSts_en'
      | sbobj.Groups.Signals(9).XData = [0 1 2 3 10 30 31 32 33 35 36]
      | sbobj.Groups.Signals(9).YData = [0 0 0 0 0 0 0 0 0 0 0]
      | sbobj.Groups.Signals(10).Name = 'V_VDS_degRdSlopeLong_s16'
      | sbobj.Groups.Signals(10).XData = [0 1 2 3 10 30 31 32 33 35 36]
      | sbobj.Groups.Signals(10).YData = [0 0 0 0 0 0 0 0 0 0 0]
      | sbobj.Groups.TimeRange = [0 36]
  V_EBR_stACCStdbySkpSts_en : Outport  Tag=STV Outport
  V_EBR_stACCBrkSkpSts_en : Outport  Tag=STV Outport  Port=2
  V_EBR_stACCHldSkpSts_en : Outport  Tag=STV Outport  Port=3
  V_EBR_stACCFalCseSts_en : Outport  Tag=STV Outport  Port=4
  V_EBR_stACCSysSts_en : Outport  Tag=STV Outport  Port=5
  V_EBR_stACCEPBSts_en : Outport  Tag=STV Outport  Port=6
  V_EBR_aACCReqValue_u16 : Outport  Tag=STV Outport  Port=7
  V_EBR_stACCSebltSts_en : Outport  Tag=STV Outport  Port=8
  V_EBR_stACCDrvrDorOpnSts_en : Outport  Tag=STV Outport  Port=9
  V_VDS_degRdSlopeLong_s16 : Outport  Tag=STV Outport  Port=10
  wires:
  Demux/1 -> V_EBR_stACCStdbySkpSts_en/1
  FromWs/1 -> Demux/1
  Demux/2 -> V_EBR_stACCBrkSkpSts_en/1
  Demux/3 -> V_EBR_stACCHldSkpSts_en/1
  Demux/4 -> V_EBR_stACCFalCseSts_en/1
  Demux/5 -> V_EBR_stACCSysSts_en/1
  Demux/6 -> V_EBR_stACCEPBSts_en/1
  Demux/7 -> V_EBR_aACCReqValue_u16/1
  Demux/8 -> V_EBR_stACCSebltSts_en/1
  Demux/9 -> V_EBR_stACCDrvrDorOpnSts_en/1
  Demux/10 -> V_VDS_degRdSlopeLong_s16/1

== system abs_CS9_LDM_w_EBRDBR/Signal Builder3 ==
  Demux : Demux  Tag=STV Demux  Outputs=2
  FromWs : FromWorkspace  Tag=STV FromWs  VariableName=tuvar  SampleTime=0  SigBuilderData=DataTag6  VnvData=DataTag7
      SigBuilderData=|
      | common.afterFinalStr = 'Extrapolate'
      | common.sampleTime = 0
      | dataSet(1).timeRange = [0 20]
      | dataSet(1).name = 'DBR_ramp'
      | dataSet(2).timeRange = [0 15]
      | dataSet(2).name = 'DBR_ramp1'
      | sbobj.Groups(1).Name = 'DBR_ramp'
      | sbobj.Groups(1).Signals(1).Name = 'Grade'
      | sbobj.Groups(1).Signals(1).XData = [0 20]
      | sbobj.Groups(1).Signals(1).YData = [0 0]
      | sbobj.Groups(1).Signals(2).Name = 'Accel_Torque'
      | sbobj.Groups(1).Signals(2).XData = [0 0.75 2 3 6.01 9.5 10 20]
      | sbobj.Groups(1).Signals(2).YData = [0 3000 5000 0 0 1200 0 0]
      | sbobj.Groups(1).TimeRange = [0 20]
      | sbobj.Groups(2).Name = 'DBR_ramp1'
      | sbobj.Groups(2).Signals(1).Name = 'Grade'
      | sbobj.Groups(2).Signals(1).XData = [0 20]
      | sbobj.Groups(2).Signals(1).YData = [0 0]
      | sbobj.Groups(2).Signals(2).Name = 'Accel_Torque'
      | sbobj.Groups(2).Signals(2).XData = [0 0.75 2 3 6.01 9.5 10 20]
      | sbobj.Groups(2).Signals(2).YData = [0 3000 3000 0 0 1200 0 0]
      | sbobj.Groups(2).TimeRange = [0 20]
  Grade : Outport  Tag=STV Outport
  Accel_Torque : Outport  Tag=STV Outport  Port=2
  wires:
  FromWs/1 -> Demux/1
  Demux/1 -> Grade/1
  Demux/2 -> Accel_Torque/1

== system abs_CS9_LDM_w_EBRDBR/Subsystem ==
  PldDist : Inport
  Minus : Sum  Inputs=+-
  Unit Delay : UnitDelay  SampleTime=-1
  Weighted Sample Time : SampleTimeMath  TsampMathOp=/
  PldSpd : Outport
  wires:
  PldDist/1 -> Minus/1, Unit Delay/1
  Weighted Sample Time/1 -> PldSpd/1
  Unit Delay/1 -> Minus/2
  Minus/1 -> Weighted Sample Time/1

== system abs_CS9_LDM_w_EBRDBR/Subsystem1 ==
  DecelReq : Inport
  Constant : Constant  Value=2
  Constant1 : Constant  Value=0
  Switch : Switch  Criteria=u2 > Threshold
  stBrkArbMode : Outport
  wires:
  Switch/1 -> stBrkArbMode/1
  DecelReq/1 -> Switch/2
  Constant/1 -> Switch/1
  Constant1/1 -> Switch/3

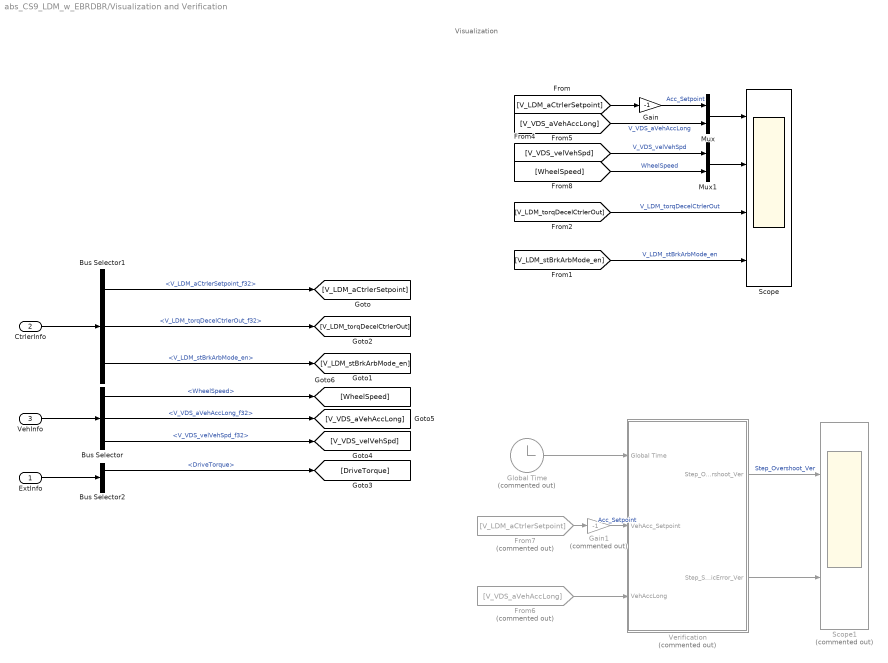
== system abs_CS9_LDM_w_EBRDBR/Visualization and Verification ==
  note: Visualization
  ExtInfo : Inport
  CtrlerInfo : Inport  Port=2
  VehInfo : Inport  Port=3
  Bus Selector : BusSelector  OutputSignals=WheelSpeed,V_VDS_aVehAccLong_f32,V_VDS_velVehSpd_f32
  Bus Selector1 : BusSelector  OutputSignals=V_LDM_aCtrlerSetpoint_f32,V_LDM_torqDecelCtrlerOut_f32,V_LDM_stBrkArbMode_en
  Bus Selector2 : BusSelector  OutputSignals=DriveTorque,Grade
  From6 : From  Commented=on  GotoTag=V_VDS_aVehAccLong
  From7 : From  Commented=on  GotoTag=V_LDM_aCtrlerSetpoint
  Gain : Gain  Gain=-1
  Gain1 : Gain  Commented=on  Gain=-1
  Global Time : Clock  Commented=on
      settings: Decimation=100
  Mux : Mux  Inputs=2
  Mux1 : Mux  Inputs=2
  Scope : Scope  NumInputPorts=4
  Scope1 : Scope  Commented=on  NumInputPorts=2
  Verification : Subsystem  Commented=on  mask{Step_Overshoot_Enable=on, Step_Overshoot_StartTime=5, Step_Overshoot_EndTime=6, Step_Overshoot_Limit=0.05, Step_StaticError_Enable=on, Step_StaticError_StartTime=5.3, Step_StaticError_EndTime=6, Step_StaticError_Limit=0.05}
      mask prompts: Step_Overshoot_Enable "Enable"; Step_Overshoot_StartTime "Start time"; Step_Overshoot_EndTime "End time"; Step_Overshoot_Limit "Upper limit"; Step_StaticError_Enable "Enable"; Step_StaticError_StartTime "Start time"; Step_StaticError_EndTime "End time"; Step_StaticError_Limit "Largest abs error"
  wires:
  Bus Selector/3 -> [V_VDS_velVehSpd]  "<V_VDS_velVehSpd_f32>"
  Mux/1 -> Scope/1
  Bus Selector/2 -> [V_VDS_aVehAccLong]  "<V_VDS_aVehAccLong_f32>"
  VehInfo/1 -> Bus Selector/1
  CtrlerInfo/1 -> Bus Selector1/1
  ExtInfo/1 -> Bus Selector2/1
  Bus Selector2/1 -> [DriveTorque]  "<DriveTorque>"
  Gain/1 -> Mux/1  "Acc_Setpoint"
  Bus Selector1/2 -> [V_LDM_torqDecelCtrlerOut]  "<V_LDM_torqDecelCtrlerOut_f32>"
  [V_LDM_torqDecelCtrlerOut] -> Scope/3  "V_LDM_torqDecelCtrlerOut"
  Bus Selector1/1 -> [V_LDM_aCtrlerSetpoint]  "<V_LDM_aCtrlerSetpoint_f32>"
  Bus Selector1/3 -> [V_LDM_stBrkArbMode_en]  "<V_LDM_stBrkArbMode_en>"
  [V_LDM_aCtrlerSetpoint] -> Gain/1
  [V_LDM_stBrkArbMode_en] -> Scope/4  "V_LDM_stBrkArbMode_en"
  [V_VDS_velVehSpd] -> Mux1/1  "V_VDS_velVehSpd"
  [V_VDS_aVehAccLong] -> Mux/2  "V_VDS_aVehAccLong"
  Global Time/1 -> Verification/1(Global Time)
  From6/1 -> Verification/3(VehAccLong)
  From7/1 -> Gain1/1
  Gain1/1 -> Verification/2(VehAcc_Setpoint)  "Acc_Setpoint"
  Verification/1(Step_Overshoot_Ver) -> Scope1/1  "Step_Overshoot_Ver"
  Verification/2(Step_StaticError_Ver) -> Scope1/2
  Bus Selector/1 -> [WheelSpeed]  "<WheelSpeed>"
  [WheelSpeed] -> Mux1/2  "WheelSpeed"
  Mux1/1 -> Scope/2

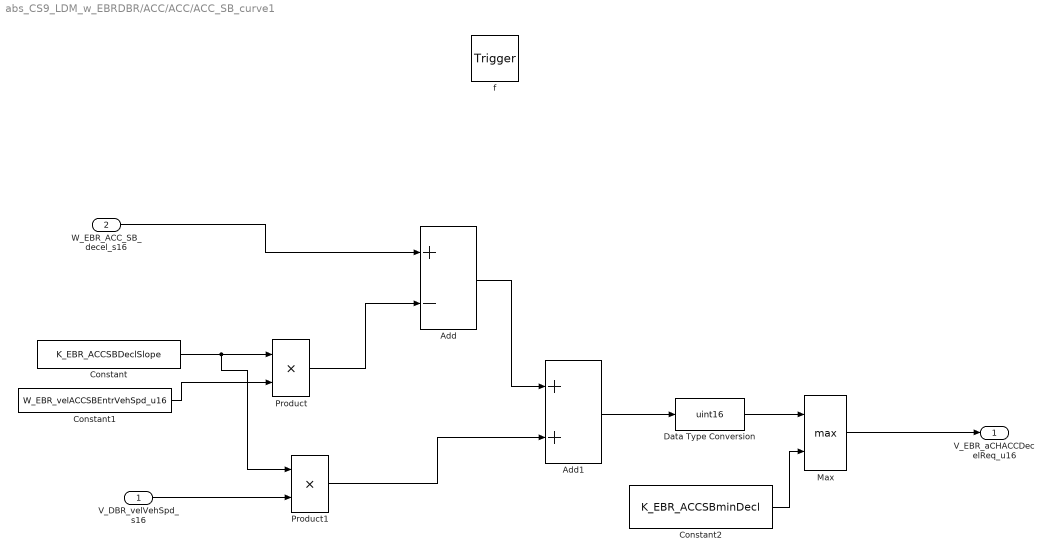
== system abs_CS9_LDM_w_EBRDBR/ACC/ACC/ACC_SB_curve1 ==
  V_DBR_velVehSpd_s16 : Inport  OutDataTypeStr=int16  PortDimensions=1
  W_EBR_ACC_SB_decel_s16 : Inport  Port=2  OutDataTypeStr=int16  PortDimensions=1
  f : TriggerPort  TriggerType=function-call  VariantControl=(inherit)
      settings: CopyFcn=Stateflow.SLINSF.SimulinkMan.removeBlockPreDeleteFcn  PreDeleteFcn=Stateflow.SLINSF.SimulinkMan.unsafePredeleteFcn
  Add : Sum  Inputs=+-
  Add1 : Sum
  Constant : Constant  Value=K_EBR_ACCSBDeclSlope
  Constant1 : Constant  Value=W_EBR_velACCSBEntrVehSpd_u16
  Constant2 : Constant  Value=K_EBR_ACCSBminDecl
  Data Type Conversion : DataTypeConversion  OutDataTypeStr=uint16
  Max : MinMax  Function=max  Inputs=2
  Product : Product
  Product1 : Product
  V_EBR_aCHACCDecelReq_u16 : Outport
  wires:
  W_EBR_ACC_SB_decel_s16/1 -> Add/1
  Constant/1 -> Product1/1, Product/1
  Constant1/1 -> Product/2
  Product/1 -> Add/2
  V_DBR_velVehSpd_s16/1 -> Product1/2
  Add/1 -> Add1/1
  Product1/1 -> Add1/2
  Add1/1 -> Data Type Conversion/1
  Data Type Conversion/1 -> Max/1
  Max/1 -> V_EBR_aCHACCDecelReq_u16/1
  Constant2/1 -> Max/2

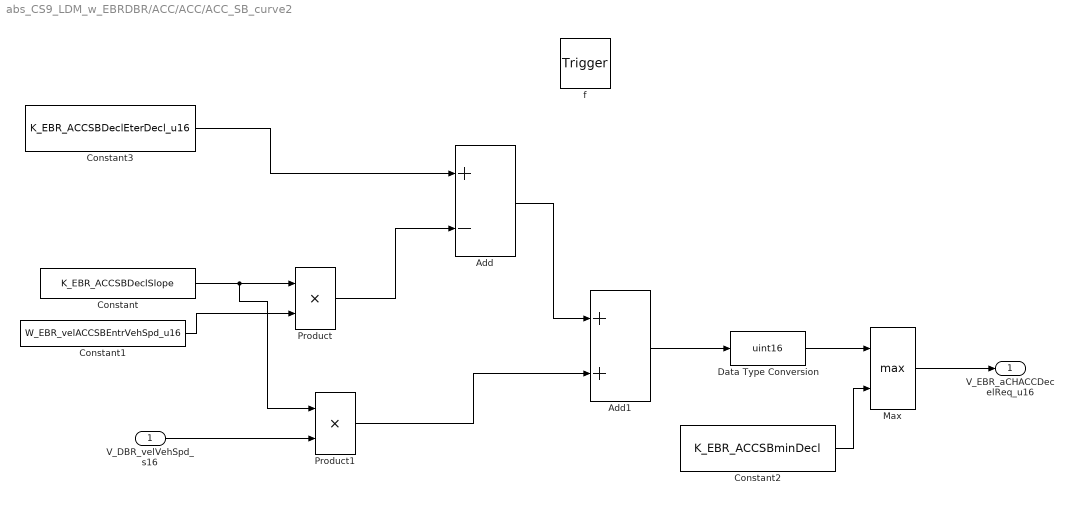
== system abs_CS9_LDM_w_EBRDBR/ACC/ACC/ACC_SB_curve2 ==
  V_DBR_velVehSpd_s16 : Inport  OutDataTypeStr=int16  PortDimensions=1
  f : TriggerPort  TriggerType=function-call  VariantControl=(inherit)
      settings: CopyFcn=Stateflow.SLINSF.SimulinkMan.removeBlockPreDeleteFcn  PreDeleteFcn=Stateflow.SLINSF.SimulinkMan.unsafePredeleteFcn
  Add : Sum  Inputs=+-
  Add1 : Sum
  Constant : Constant  Value=K_EBR_ACCSBDeclSlope
  Constant1 : Constant  Value=W_EBR_velACCSBEntrVehSpd_u16
  Constant2 : Constant  Value=K_EBR_ACCSBminDecl
  Constant3 : Constant  Value=K_EBR_ACCSBDeclEterDecl_u16
  Data Type Conversion : DataTypeConversion  OutDataTypeStr=uint16
  Max : MinMax  Function=max  Inputs=2
  Product : Product
  Product1 : Product
  V_EBR_aCHACCDecelReq_u16 : Outport
  wires:
  Constant2/1 -> Max/2
  Data Type Conversion/1 -> Max/1
  Constant1/1 -> Product/2
  Add1/1 -> Data Type Conversion/1
  Constant/1 -> Product1/1, Product/1
  V_DBR_velVehSpd_s16/1 -> Product1/2
  Constant3/1 -> Add/1
  Product/1 -> Add/2
  Product1/1 -> Add1/2
  Add/1 -> Add1/1
  Max/1 -> V_EBR_aCHACCDecelReq_u16/1

== system abs_CS9_LDM_w_EBRDBR/ACC/ACC/ACC_hold_curve ==
  V_VDS_degRdSlopeLong_s16 : Inport  OutDataTypeStr=int16  PortDimensions=1
  f : TriggerPort  TriggerType=function-call  VariantControl=(inherit)
      settings: CopyFcn=Stateflow.SLINSF.SimulinkMan.removeBlockPreDeleteFcn  PreDeleteFcn=Stateflow.SLINSF.SimulinkMan.unsafePredeleteFcn
  Abs : Abs
  Constant : Constant  Value=1000  OutDataTypeStr=int16
  Constant1 : Constant  Value=K_EBR_aACCHold_flat_u16
  Constant2 : Constant  Value=10  OutDataTypeStr=int16
  Data Type Conversion : DataTypeConversion  OutDataTypeStr=uint16
  Divide : Product  Inputs=*/
  Product : Product
  Sum : Sum  Inputs=|++
  Trigonometric Function : Trigonometry  ApproximationMethod=CORDIC
  V_EBR_aCHACCDecelReq_u16 : Outport
  wires:
  V_VDS_degRdSlopeLong_s16/1 -> Abs/1
  Abs/1 -> Divide/1
  Divide/1 -> Trigonometric Function/1
  Trigonometric Function/1 -> Product/1
  Constant/1 -> Product/2
  Product/1 -> Sum/1
  Sum/1 -> Data Type Conversion/1
  Constant1/1 -> Sum/2
  Constant2/1 -> Divide/2
  Data Type Conversion/1 -> V_EBR_aCHACCDecelReq_u16/1

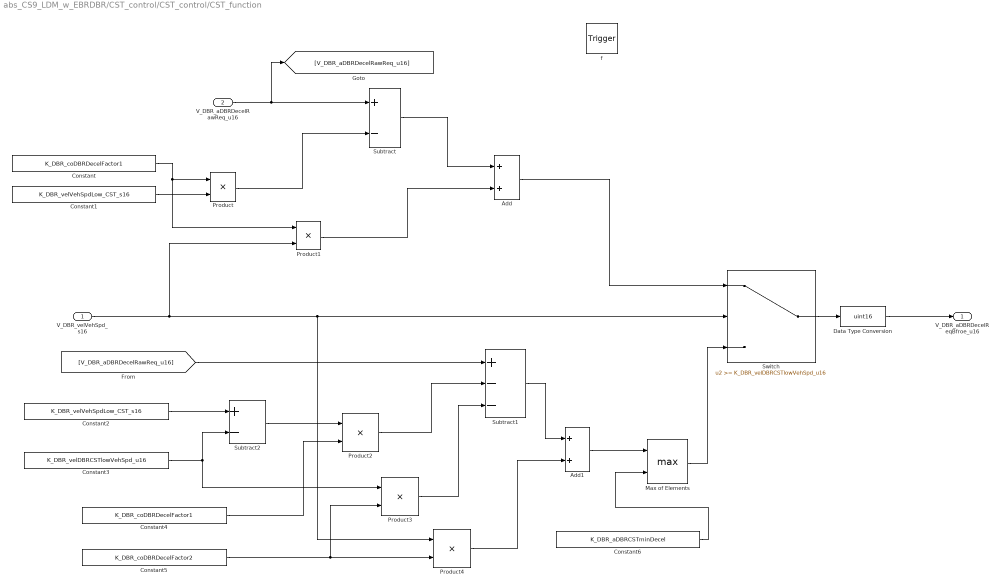
== system abs_CS9_LDM_w_EBRDBR/CST_control/CST_control/CST_function ==
  V_DBR_velVehSpd_s16 : Inport  OutDataTypeStr=int16  PortDimensions=1
  V_DBR_aDBRDecelRawReq_u16 : Inport  Port=2  OutDataTypeStr=uint16  PortDimensions=1
  f : TriggerPort  TriggerType=function-call  VariantControl=(inherit)
      settings: CopyFcn=Stateflow.SLINSF.SimulinkMan.removeBlockPreDeleteFcn  PreDeleteFcn=Stateflow.SLINSF.SimulinkMan.unsafePredeleteFcn
  Add : Sum
  Add1 : Sum
  Constant : Constant  Value=K_DBR_coDBRDecelFactor1
  Constant1 : Constant  Value=K_DBR_velVehSpdLow_CST_s16
  Constant2 : Constant  Value=K_DBR_velVehSpdLow_CST_s16
  Constant3 : Constant  Value=K_DBR_velDBRCSTlowVehSpd_u16
  Constant4 : Constant  Value=K_DBR_coDBRDecelFactor1
  Constant5 : Constant  Value=K_DBR_coDBRDecelFactor2
  Constant6 : Constant  Value=K_DBR_aDBRCSTminDecel
  Data Type Conversion : DataTypeConversion  OutDataTypeStr=uint16
  Max of Elements : MinMax  Function=max  Inputs=2
  Product{,1..4} (5 alike) : Product
  Subtract : Sum  Inputs=+-
  Subtract1 : Sum  Inputs=+--
  Subtract2 : Sum  Inputs=+-
  Switch : Switch  Threshold=K_DBR_velDBRCSTlowVehSpd_u16
  V_DBR_aDBRDecelReqBfroe_u16 : Outport
  wires:
  Switch/1 -> Data Type Conversion/1
  Data Type Conversion/1 -> V_DBR_aDBRDecelReqBfroe_u16/1
  V_DBR_aDBRDecelRawReq_u16/1 -> [V_DBR_aDBRDecelRawReq_u16], Subtract/1
  V_DBR_velVehSpd_s16/1 -> Product1/2, Product4/1, Switch/2
  Subtract/1 -> Add/1
  Add/1 -> Switch/1
  Product1/1 -> Add/2
  Constant/1 -> Product1/1, Product/1
  Constant1/1 -> Product/2
  Product/1 -> Subtract/2
  [V_DBR_aDBRDecelRawReq_u16] -> Subtract1/1
  Constant2/1 -> Subtract2/1
  Constant3/1 -> Subtract2/2, Product3/1
  Subtract2/1 -> Product2/1
  Constant4/1 -> Product2/2
  Constant5/1 -> Product4/2, Product3/2
  Product2/1 -> Subtract1/2
  Product3/1 -> Subtract1/3
  Subtract1/1 -> Add1/1
  Product4/1 -> Add1/2
  Add1/1 -> Max of Elements/1
  Max of Elements/1 -> Switch/3
  Constant6/1 -> Max of Elements/2

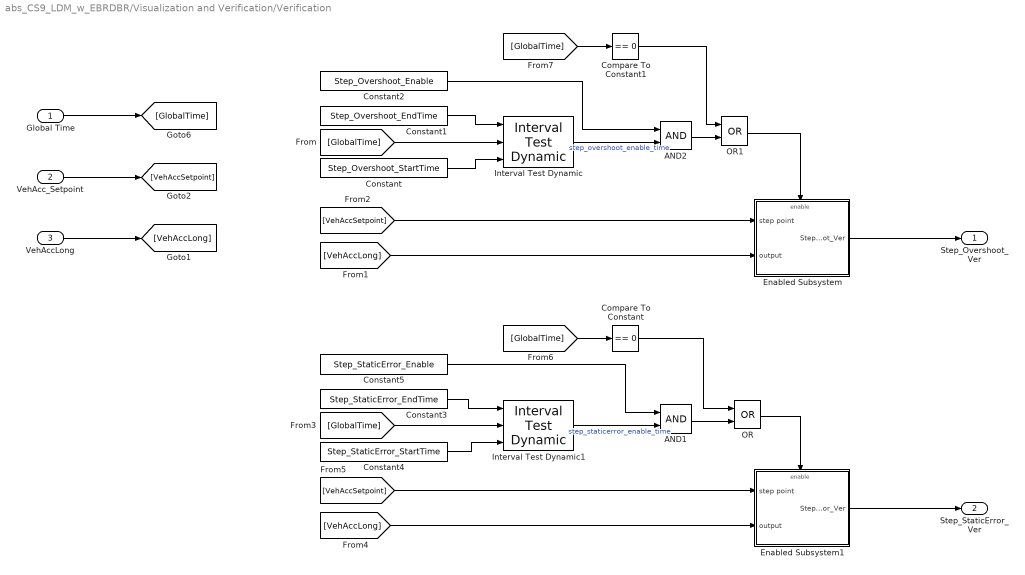
== system abs_CS9_LDM_w_EBRDBR/Visualization and Verification/Verification ==
  Global Time : Inport
  VehAcc_Setpoint : Inport  Port=2
  VehAccLong : Inport  Port=3
  AND1 : Logic  AllPortsSameDT=off  OutDataTypeStr=boolean
  AND2 : Logic  AllPortsSameDT=off  OutDataTypeStr=boolean
  Compare To Constant : simulink/Logic and Bit Operations/Compare To Constant  relop===  const=0  OutDataTypeStr=boolean
  Compare To Constant1 : simulink/Logic and Bit Operations/Compare To Constant  relop===  const=0  OutDataTypeStr=boolean
  Constant : Constant  Value=Step_Overshoot_StartTime
  Constant1 : Constant  Value=Step_Overshoot_EndTime
  Constant2 : Constant  Value=Step_Overshoot_Enable
  Constant3 : Constant  Value=Step_StaticError_EndTime
  Constant4 : Constant  Value=Step_StaticError_StartTime
  Constant5 : Constant  Value=Step_StaticError_Enable
  Enabled Subsystem : Subsystem  TreatAsAtomicUnit=on
  Enabled Subsystem1 : Subsystem  TreatAsAtomicUnit=on
  Interval Test Dynamic : simulink/Logic and Bit Operations/Interval Test Dynamic  IntervalClosedRight=off  IntervalClosedLeft=off  OutDataTypeStr=boolean
      settings: SourceProductBaseCode=SL
  Interval Test Dynamic1 : simulink/Logic and Bit Operations/Interval Test Dynamic  IntervalClosedRight=off  IntervalClosedLeft=off  OutDataTypeStr=boolean
      settings: SourceProductBaseCode=SL
  OR : Logic  Operator=OR  AllPortsSameDT=off  OutDataTypeStr=boolean
  OR1 : Logic  Operator=OR  AllPortsSameDT=off  OutDataTypeStr=boolean
  Step_Overshoot_Ver : Outport
  Step_StaticError_Ver : Outport  Port=2
  wires:
  Global Time/1 -> [GlobalTime]
  [GlobalTime] -> Interval Test Dynamic/2
  Constant1/1 -> Interval Test Dynamic/1
  VehAccLong/1 -> [VehAccLong]
  Interval Test Dynamic/1 -> AND2/2  "step_overshoot_enable_time"
  Constant/1 -> Interval Test Dynamic/3
  Enabled Subsystem/1(Step_Overshoot_Ver) -> Step_Overshoot_Ver/1
  [VehAccLong] -> Enabled Subsystem/2(output)
  VehAcc_Setpoint/1 -> [VehAccSetpoint]
  [VehAccSetpoint] -> Enabled Subsystem/1(step point)
  Constant2/1 -> AND2/1
  OR1/1 -> Enabled Subsystem/Enable
  Enabled Subsystem1/1(Step_StaticError_Ver) -> Step_StaticError_Ver/1
  Constant5/1 -> AND1/1
  Constant4/1 -> Interval Test Dynamic1/3
  Interval Test Dynamic1/1 -> AND1/2  "step_staticerror_enable_time"
  [VehAccSetpoint] -> Enabled Subsystem1/1(step point)
  Constant3/1 -> Interval Test Dynamic1/1
  [GlobalTime] -> Interval Test Dynamic1/2
  [VehAccLong] -> Enabled Subsystem1/2(output)
  AND1/1 -> OR/2
  [GlobalTime] -> Compare To Constant/1
  Compare To Constant/1 -> OR/1
  OR/1 -> Enabled Subsystem1/Enable
  Compare To Constant1/1 -> OR1/1
  [GlobalTime] -> Compare To Constant1/1
  AND2/1 -> OR1/2

== system abs_CS9_LDM_w_EBRDBR/Visualization and Verification/Verification/Enabled Subsystem ==
  note: accel: positive
      | decel: negative
  step point : Inport
  output : Inport  Port=2
  Enable : EnablePort  StatesWhenEnabling=reset
  Check Dynamic  Upper Bound : simulink/Model Verification/Check Dynamic  Upper Bound  Description=u < max  enabled=on  stopWhenAssertionFail=off  export=on  icon=graphic
      settings: SourceProductBaseCode=SL
  Constant1 : Constant  Value=Step_Overshoot_Limit
  Minus : Sum  Inputs=+-
  Step_Overshoot_Ver : Outport
  wires:
  step point/1 -> Minus/1
  output/1 -> Minus/2
  Minus/1 -> Check Dynamic  Upper Bound/2
  Check Dynamic  Upper Bound/1 -> Step_Overshoot_Ver/1
  Constant1/1 -> Check Dynamic  Upper Bound/1

== system abs_CS9_LDM_w_EBRDBR/Visualization and Verification/Verification/Enabled Subsystem1 ==
  note: accel: positive
      | decel: negative
  step point : Inport
  output : Inport  Port=2
  Enable : EnablePort  StatesWhenEnabling=reset
  Abs : Abs
  Check  Dynamic Range : simulink/Model Verification/Check  Dynamic Range  Description=min < u < max  enabled=on  stopWhenAssertionFail=off  export=on  icon=graphic
      settings: SourceProductBaseCode=SL
  Constant1 : Constant  Value=Step_StaticError_Limit
  Gain : Gain  Gain=-1
  Minus : Sum  Inputs=+-
  Step_StaticError_Ver : Outport
  wires:
  step point/1 -> Minus/1
  output/1 -> Minus/2
  Minus/1 -> Check  Dynamic Range/3
  Check  Dynamic Range/1 -> Step_StaticError_Ver/1
  Constant1/1 -> Abs/1
  Gain/1 -> Check  Dynamic Range/2
  Abs/1 -> Gain/1, Check  Dynamic Range/1

== stateflow chart CST_control/CST_control ==
  state control_initial
    en,du:
    V_DBR_stDBRCSTRunbleSts_en=DBRCSTRunbleSts_en_t.initial;
  state standstill_control
    en,du:
    V_DBR_stDBRCSTRunbleSts_en=DBRCSTRunbleSts_en_t.standstill_control;
    standstill_control -> (junction 12) [order 1]
    (junction 12) -> (junction 13) [order 1] : [V_DBR_lenPdlDist_s16<=K_DBR_lenDBRStdlstlDegdlvl_u16]
    (junction 12) -> (junction 14) [order 2]
    (junction 13) -> (junction 15) : {V_DBR_aDBRDecelReqBfroe_u16=min(V_DBR_aDBRDecelRawReq_u16,K_DBR_aDBRDecelStdlstlDegdlvl1_u16);}
    (junction 14) -> (junction 15) : {V_DBR_aDBRDecelReqBfroe_u16=min(V_DBR_aDBRDecelRawReq_u16,K_DBR_aDBRDecelStdlstlDegdlvl2_u16);}
  state dynamic_control
    en,du:
    V_DBR_aDBRDecelReqBfroe_u16=V_DBR_aDBRDecelRawReq_u16;
    V_DBR_stDBRCSTRunbleSts_en=DBRCSTRunbleSts_en_t.dynamic_control;
  state V_DBR_aDBRDecelReqBfroe_u16=CST_function(V_DBR_velVehSpd_s16,V_DBR_aDBRDecelRawReq_u16) [function]
  state CST_control
    state CST_standby
      CST_standby -> (junction 32) [order 1]
      (junction 32) -> (junction 33) [order 1] : [V_EBR_stACCVehSpdLvl_en==ACCVehSpdLvl_en_t.standstill]
      (junction 32) -> (junction 34) [order 2]
      (junction 33) -> (junction 35) : {V_DBR_stDBRCSTRunbleSts_en=DBRCSTRunbleSts_en_t.CST_standby_standstill_control;}
      (junction 35) -> (junction 36) [order 1] : [V_DBR_lenPdlDist_s16<=K_DBR_lenDBRStdlstlDegdlvl_u16]
      (junction 34) -> (junction 37) : {V_DBR_stDBRCSTRunbleSts_en=DBRCSTRunbleSts_en_t.CST_standby_dynamic_control;}
      (junction 35) -> (junction 38) [order 2]
      (junction 36) -> (junction 39) : {V_DBR_aDBRDecelReqBfroe_u16=min(V_DBR_aDBRDecelRawReq_u16,K_DBR_aDBRDecelStdlstlDegdlvl1_u16);}
      (junction 37) -> (junction 40)
      (junction 38) -> (junction 39) : {V_DBR_aDBRDecelReqBfroe_u16=min(V_DBR_aDBRDecelRawReq_u16,K_DBR_aDBRDecelStdlstlDegdlvl2_u16);}
      (junction 39) -> (junction 41)
      (junction 40) -> (junction 41) : {V_DBR_aDBRDecelReqBfroe_u16=V_DBR_aDBRDecelRawReq_u16;}
    state CST_off
      V_DBR_stDBRCSTRunbleSts_en=DBRCSTRunbleSts_en_t.CST_off;
      CST_off -> (junction 54) [order 1]
      (junction 54) -> (junction 55) [order 1] : [V_DBR_lenPdlDist_s16<=K_DBR_lenDBRStdlstlDegdlvl_u16]
      (junction 54) -> (junction 56) [order 2]
      (junction 55) -> (junction 57) : {V_DBR_aDBRDecelReqBfroe_u16=min(V_DBR_aDBRDecelRawReq_u16,K_DBR_aDBRDecelStdlstlDegdlvl1_u16);}
      (junction 56) -> (junction 57) : {V_DBR_aDBRDecelReqBfroe_u16=min(V_DBR_aDBRDecelRawReq_u16,K_DBR_aDBRDecelStdlstlDegdlvl2_u16);}
    state CST_active
      en,du:
      V_DBR_aDBRDecelReqBfroe_u16=CST_function(V_DBR_velVehSpd_s16,V_DBR_aDBRDecelRawReq_u16);
      V_DBR_stDBRCSTRunbleSts_en=DBRCSTRunbleSts_en_t.CST_active;
    state CST_emergency_control
      en,du:
      V_DBR_aDBRDecelReqBfroe_u16=V_DBR_aDBRDecelRawReq_u16;
      V_DBR_stDBRCSTRunbleSts_en=DBRCSTRunbleSts_en_t.CST_emergency_control;
    (default) -> CST_standby
    CST_standby -> CST_active [order 1] : [(V_DBR_velVehSpd_s16<=K_DBR_velVehSpdLow_CST_s16...
        | &&V_DBR_velVehSpd_s16>int16(0))...
        | &&(V_DBR_aDBRDecelRawReq_u16<K_DBR_aDBRDecelEmgHigh_CST_u16...
        | &&V_DBR_aDBRDecelRawReq_u16>=K_DBR_aDBRDecelSftLow_CST_u16)...
        | &&V_DBR_blCSTPreCdtin_bl==true]
    CST_off -> CST_standby [order 1] : [K_DBR_blCSTSwch_bl==false || V_DBR_blCSTSysFail_bl==true||V_DBR_stPdlAply_bl==false]
    CST_active -> CST_standby [order 1] : [V_DBR_blAYCA_bl==true||V_DBR_blABSA_bl==true||...
        | V_DBR_blTCSA_bl==true||V_DBR_stPdlAply_bl==false...
        | ||K_DBR_blCSTSwch_bl==false || V_DBR_blCSTSysFail_bl==true]
    CST_emergency_control -> CST_standby [order 2] : [K_DBR_blCSTSwch_bl==false || V_DBR_blCSTSysFail_bl==true||V_DBR_stPdlAply_bl==false]
    CST_active -> CST_off [order 3] : [V_EBR_stACCVehSpdLvl_en==ACCVehSpdLvl_en_t.standstill]
    CST_active -> CST_emergency_control [order 2] : [V_DBR_velPdlDistSpd_s16>=K_DBR_velCSTPdlDistSpdLmt_s16||V_DBR_aDBRDecelRawReq_u16>=K_DBR_aDBRDecelEmgHigh_CST_u16||V_DBR_blLosDecel_bl==true]
    CST_emergency_control -> CST_off [order 1] : [V_EBR_stACCVehSpdLvl_en==ACCVehSpdLvl_en_t.standstill]
  (default) -> control_initial
  control_initial -> dynamic_control [order 2] : [V_EBR_stACCVehSpdLvl_en~=ACCVehSpdLvl_en_t.standstill]
  control_initial -> standstill_control [order 1] : [V_EBR_stACCVehSpdLvl_en==ACCVehSpdLvl_en_t.standstill]
  standstill_control -> dynamic_control [order 1] : [V_EBR_stACCVehSpdLvl_en~=ACCVehSpdLvl_en_t.standstill]
  dynamic_control -> standstill_control [order 1] : [V_EBR_stACCVehSpdLvl_en==ACCVehSpdLvl_en_t.standstill]
  dynamic_control -> CST_control [order 2] : [K_DBR_blCSTSwch_bl==true&&V_DBR_blCSTSysFail_bl==false]
  CST_control -> dynamic_control [order 2] : [(K_DBR_blCSTSwch_bl==false || V_DBR_blCSTSysFail_bl==true)&&V_EBR_stACCVehSpdLvl_en~=ACCVehSpdLvl_en_t.standstill]
  standstill_control -> CST_control [order 2] : [K_DBR_blCSTSwch_bl==true&&V_DBR_blCSTSysFail_bl==false]
  CST_control -> standstill_control [order 1] : [(K_DBR_blCSTSwch_bl==false || V_DBR_blCSTSysFail_bl==true)&&V_EBR_stACCVehSpdLvl_en==ACCVehSpdLvl_en_t.standstill]
  data: V_DBR_velVehSpd_s16 function_input int16 size=1; V_DBR_aDBRDecelRawReq_u16 function_input uint16 size=1; V_DBR_aDBRDecelReqBfroe_u16 function_output double; V_EBR_stACCVehSpdLvl_en input Enum: ACCVehSpdLvl_en_t; V_DBR_velVehSpd_s16 input int16; V_DBR_aDBRDecelRawReq_u16 input uint16; V_DBR_stPdlAply_bl input boolean; V_DBR_blCSTPreCdtin_bl input boolean; V_DBR_blAYCA_bl input boolean; V_DBR_blABSA_bl input boolean; V_DBR_blTCSA_bl input boolean; V_DBR_blCSTSysFail_bl input boolean; V_DBR_blLosDecel_bl input boolean; V_DBR_lenPdlDist_s16 input int16; V_DBR_aDBRDecelReqBfroe_u16 output uint16; V_DBR_stDBRCSTRunbleSts_en output Enum: DBRCSTRunbleSts_en_t; K_DBR_velVehSpdLow_CST_s16 parameter double; K_DBR_aDBRDecelEmgHigh_CST_u16 parameter double; K_DBR_aDBRDecelSftLow_CST_u16 parameter double; K_DBR_blCSTSwch_bl parameter double; K_DBR_aDBRDecelStdlstlDegdlvl2_u16 parameter double; K_DBR_aDBRDecelStdlstlDegdlvl1_u16 parameter double; K_DBR_lenDBRStdlstlDegdlvl_u16 parameter double; V_DBR_velPdlDistSpd_s16 input int16; K_DBR_velCSTPdlDistSpdLmt_s16 parameter double
